simulink model "model_luz"  (R2021b)
settings: Solver=VariableStepAuto  StartTime=0.0  StopTime=T  MaxStep=1e-3  RelTol=1e-3
undefined symbols (not defined in the file): J, Mf
settings Model: Creator=mateusz  LastModifiedBy=mateusz
settings SolverCC: MaxConsecutiveMinStep=10000  ZeroCrossControl=EnableAll  ZeroCrossAlgorithm=Adaptive
settings DebuggingCC: IgnoredZcDiagnostic=none

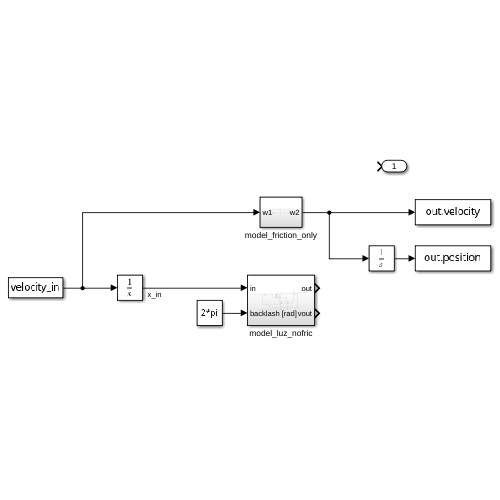
[thumbnail: Simulink's stored preview of the top-level diagram]
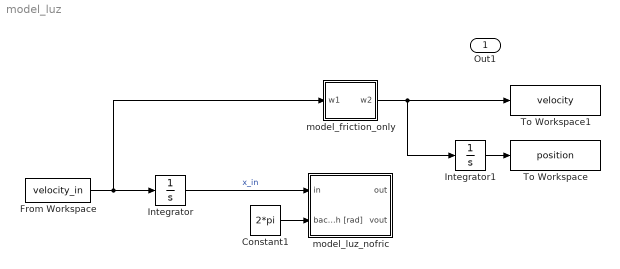
== system model_luz ==
  Constant1 : Constant  Value=2*pi
  From Workspace : FromWorkspace  VariableName=velocity_in
  Integrator : Integrator
  Integrator1 : Integrator
  To Workspace : ToWorkspace  VariableName=position  SaveFormat=Structure With Time  SampleTime=-1
  To Workspace1 : ToWorkspace  VariableName=velocity  SaveFormat=Structure With Time  SampleTime=-1
  model_friction_only : Subsystem
  model_luz_nofric : Subsystem
  Out1 : Outport
  wires:
  Constant1/1 -> model_luz_nofric/2(backlash [rad])
  Integrator/1 -> model_luz_nofric/1(in)  "x_in"
  From Workspace/1 -> model_friction_only/1(w1), Integrator/1
  model_friction_only/1(w2) -> To Workspace1/1, Integrator1/1
  Integrator1/1 -> To Workspace/1

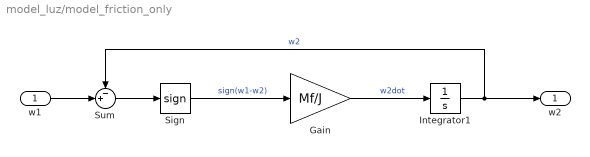
== system model_luz/model_friction_only ==
  w1 : Inport
  Gain : Gain  Gain=Mf/J
  Integrator1 : Integrator
  Sign : Signum
  Sum : Sum  Inputs=-+|
  w2 : Outport
  wires:
  Sum/1 -> Sign/1
  Gain/1 -> Integrator1/1  "w2dot"
  Integrator1/1 -> w2/1, Sum/1  "w2"
  Sign/1 -> Gain/1  "sign(w1-w2)"
  w1/1 -> Sum/2

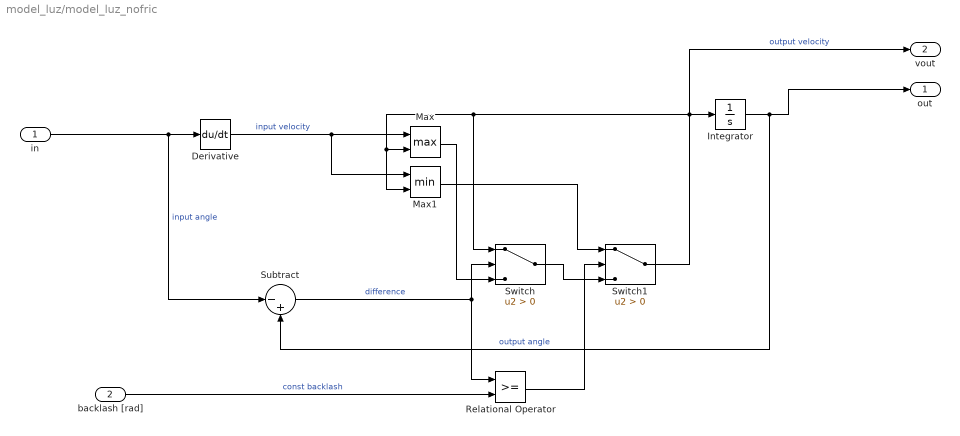
== system model_luz/model_luz_nofric ==
  in : Inport
  backlash [rad] : Inport  Port=2
  Derivative : Derivative
  Integrator : Integrator
  Max : MinMax  Function=max  Inputs=2
  Max1 : MinMax  Inputs=2
  Relational Operator : RelationalOperator  OutDataTypeStr=boolean  RndMeth=Simplest
  Subtract : Sum  Inputs=|-+
  Switch : Switch  Criteria=u2 > Threshold
  Switch1 : Switch  Criteria=u2 > Threshold
  out : Outport
  vout : Outport  Port=2
  wires:
  Switch/1 -> Switch1/3
  Max/1 -> Switch/3
  Switch1/1 -> Switch/1, Max1/2, Max/2, vout/1, Integrator/1  "output velocity"
  Max1/1 -> Switch1/1
  Subtract/1 -> Relational Operator/1, Switch/2  "difference"
  Derivative/1 -> Max1/1, Max/1  "input velocity"
  in/1 -> Subtract/1, Derivative/1  "input angle"
  Integrator/1 -> out/1, Subtract/2  "output angle"
  backlash [rad]/1 -> Relational Operator/2  "const backlash"
  Relational Operator/1 -> Switch1/2
